simulink subsystem "springLookup_mdl"  (R2023a)
settings: Solver=VariableStepAuto  StartTime=0.0  StopTime=10.0  RelTol=1e-3
undefined symbols (not defined in the file): obj
settings Model: Creator=grouleau  LastModifiedBy=grouleau

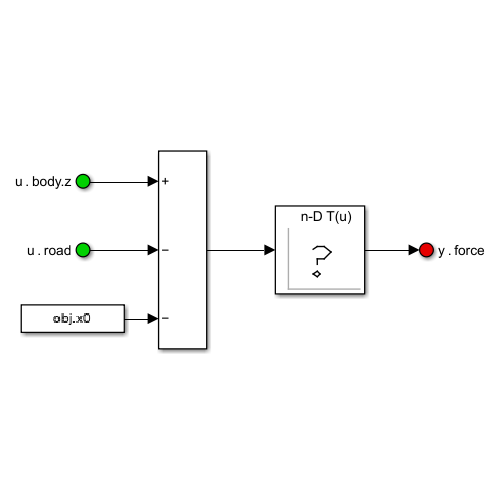
[thumbnail: Simulink's stored preview of the top-level diagram]
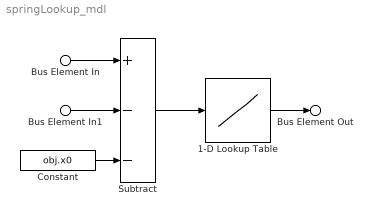
== system springLookup_mdl ==
  Bus Element In : Inport  PortName=u  Element=body.z
  Bus Element In1 : Inport  PortName=u  Element=road
  1-D Lookup Table : Lookup_n-D  NumberOfTableDimensions=1  BreakpointsForDimension1=obj.x  Table=obj.K  InternalRulePriority=Speed  RndMeth=Simplest
  Constant : Constant  Value=obj.x0
  Subtract : Sum  Inputs=+--
  Bus Element Out : Outport  PortName=y  Element=force
  wires:
  Bus Element In/1 -> Subtract/1
  Bus Element In1/1 -> Subtract/2
  Constant/1 -> Subtract/3
  Subtract/1 -> 1-D Lookup Table/1
  1-D Lookup Table/1 -> Bus Element Out/1
